simulink model "chap2_1sim"  (R2025b)
settings: Solver=FixedStepAuto  StartTime=0.0  StopTime=1  FixedStep=0.001  RelTol=1e-3  EnableMultiTasking=on
settings Model: ExtModeTrigMode=oneshot  ExtModeArmWhenConnect=off  Creator=J  LastModifiedBy=J
settings DataIOCC: SaveFormat=Array  SignalLoggingSaveFormat=ModelDataLogs  ReturnWorkspaceOutputs=off  SignalLoggingName=sigsOut
settings OptimizationCC: BooleanDataType=off  ReuseModelBlockBuffer=off
settings DebuggingCC: SaveWithParameterizedLinksMsg=none  UnderspecifiedInitializationDetection=Classic  MergeDetectMultiDrivingBlocksExec=none  SignalResolutionControl=TryResolveAllWithWarning  MultiTaskDSMMsg=warning  MultiTaskCondExecSysMsg=none  UnconnectedInputMsg=warning  UnconnectedOutputMsg=warning  UnconnectedLineMsg=warning
settings HardwareCC: ProdBitPerPointer=32.0  ProdBitPerSizeT=32.0  ProdBitPerPtrDiffT=32.0  ProdLargestAtomicFloat=None  ProdIntDivRoundTo=Undefined  ProdEndianess=Unspecified  ProdWordSize=32.0  ProdHWDeviceType=32-bit Generic  TargetUnknown=on
settings ModelReferenceCC: PropagateSignalLabelsOutOfModel=off
settings RTWCC: GPUComputeCapability=3.5
settings GRTTargetCC: CombineOutputUpdateFcns=off  GRTInterface=on
settings ConfigComp: CovMetricSettings=dw  CovSaveCumulativeToWorkspaceVar=on  CovSaveSingleToWorkspaceVar=on
settings SimscapeCC: SimscapeLogDecimation=1  SimscapeLogDataHistory=5000

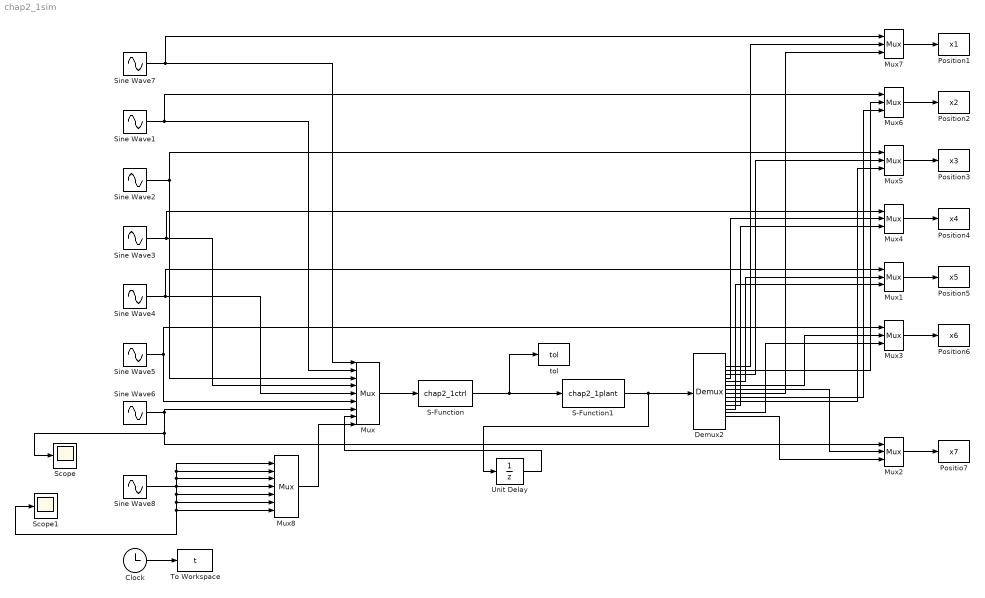
== system chap2_1sim ==
  Clock : Clock
  Demux2 : Demux  Outputs=14
      settings: DisplayOption=none
  Mux : Mux  Inputs=9
  Mux{1..7} (7 alike) : Mux  Inputs=3
  Mux8 : Mux  Inputs=7
  Positio7 : ToWorkspace  VariableName=x7  SampleTime=-1
  Position1 : ToWorkspace  VariableName=x1  SampleTime=-1
  Position2 : ToWorkspace  VariableName=x2  SampleTime=-1
  Position3 : ToWorkspace  VariableName=x3  SampleTime=-1
  Position4 : ToWorkspace  VariableName=x4  SampleTime=-1
  Position5 : ToWorkspace  VariableName=x5  SampleTime=-1
  Position6 : ToWorkspace  VariableName=x6  SampleTime=-1
  S-Function : S-Function  FunctionName=chap2_1ctrl  SFunctionDeploymentMode=off  EnableBusSupport=off
  S-Function1 : S-Function  FunctionName=chap2_1plant  SFunctionDeploymentMode=off  EnableBusSupport=off
  Scope : Scope
      settings: ActiveDisplayYMinimum=-1  ActiveDisplayYMaximum=1
  Scope1 : Scope
  Sine Wave{1..7} (7 alike) : Sin  SampleTime=0
  Sine Wave8 : Sin  Phase=pi/2  SampleTime=0
  To Workspace : ToWorkspace  VariableName=t  SampleTime=-1
  Unit Delay : UnitDelay  SampleTime=-1  HasFrameUpgradeWarning=on
  tol : ToWorkspace  VariableName=tol  SampleTime=-1
  wires:
  Mux/1 -> S-Function/1
  Mux2/1 -> Positio7/1
  Mux3/1 -> Position6/1
  Clock/1 -> To Workspace/1
  Mux1/1 -> Position5/1
  Mux4/1 -> Position4/1
  Mux5/1 -> Position3/1
  Mux6/1 -> Position2/1
  Mux7/1 -> Position1/1
  S-Function1/1 -> Unit Delay/1, Demux2/1
  Sine Wave7/1 -> Mux/1, Mux7/1
  Demux2/1 -> Mux7/2
  Demux2/2 -> Mux6/2
  Demux2/3 -> Mux5/2
  Demux2/4 -> Mux4/2
  Demux2/5 -> Mux1/2
  Demux2/6 -> Mux3/2
  Demux2/7 -> Mux2/2
  Demux2/8 -> Mux7/3
  Demux2/9 -> Mux6/3
  Demux2/10 -> Mux5/3
  Demux2/11 -> Mux4/3
  Demux2/12 -> Mux1/3
  Demux2/13 -> Mux3/3
  Demux2/14 -> Mux2/3
  Sine Wave1/1 -> Mux/2, Mux6/1
  Sine Wave2/1 -> Mux/3, Mux5/1
  Sine Wave3/1 -> Mux/4, Mux4/1
  Sine Wave4/1 -> Mux/5, Mux1/1
  Sine Wave5/1 -> Mux/6, Mux3/1
  Sine Wave6/1 -> Scope/1, Mux2/1, Mux/7
  Sine Wave8/1 -> Scope1/1, Mux8/7, Mux8/6, Mux8/5, Mux8/1, Mux8/2, Mux8/3, Mux8/4
  Mux8/1 -> Mux/9
  S-Function/1 -> S-Function1/1, tol/1
  Unit Delay/1 -> Mux/8
